simulink model "LKAS_AutoSave_DF_20220408_1006_SW62"  (R2018b)
settings: Solver=FixedStepDiscrete  StartTime=0.0  StopTime=10.0  FixedStep=0.01  RelTol=1e-3
undefined symbols (not defined in the file): LKA_CarWidth, LKA_SampleTime, LKA_StrRatio_C, LKA_Veh2CamL_C, LKA_Veh2CamW_C, LKA_WhlBaseL_C, LL_CompHdAg_C, LL_CompSWA_C, LL_CrvtPrvwT_C, LL_DesDvt_C, LL_DvtComp_C, LL_DvtPrvwT_C, LL_DvtSpdDet_vDvtSpdMin_C, LL_HandsOff_ExitTime, LL_HandsOff_TextTime, LL_HandsOff_WarnTime, LL_HdAgExT_C, LL_HdAgPrvwT_C, LL_LAccMax_C, LL_LAccRMax_C, LL_LDW_EarliestWarnLine_C, LL_LDW_LatestWarnLine_C, LL_LDWS_SUPPRESS_HEADING, LL_LFClb_TFC_FfCtlRatio_C, LL_LFClb_TFC_KdBalance_C, LL_LFClb_TFC_KdMaxSWA_C, LL_LFClb_TFC_KdV1_C, LL_LFClb_TFC_KdV2_C, LL_LFClb_TFC_KdVehSpdLwr_C, LL_LFClb_TFC_KdVehSpdUpr_C, LL_LFClb_TFC_Ki_C, LL_LFClb_TFC_KiMaxSWA_C, LL_LFClb_TFC_Kp_C, LL_LFClb_TFC_KpKlat_C, LL_LFClb_TFC_KpV1_C, LL_LFClb_TFC_KpV2_C, LL_LFClb_TFC_KpVehSpdLwr_C, LL_LFClb_TFC_KpVehSpdUpr_C, LL_LFClb_TFC_PrvwT_C, LL_LKA_EarliestWarnLine_C, LL_LKA_LatestWarnLine_C, LL_LKAExPrcs_ExitC0Dvt, LL_LKAExPrcs_ExitC0Swt, LL_LKAExPrcs_tiExitDelayTime3, LL_LKAExPrcs_tiExitTime1, LL_LKAExPrcs_tiExitTime2, LL_LKAExPrcs_tiExitTime3, LL_LKAS_OUT_OF_CONTROL_LAT_VEL, LL_LKAS_OUT_OF_CONTROL_TTLC, LL_LKASWASyn_M0, LL_LKASWASyn_M1, LL_LKASWASyn_M2, LL_LKASWASyn_M3D, LL_LKASWASyn_M3K_DT, LL_LKASWASyn_M3K_MSD, LL_LKASWASyn_M4K, LL_LKASWASyn_SWAaddMax, LL_LKASWASyn_T2, LL_LKASWASyn_tiTrqSwaRtTime, LL_LKASWASyn_tiTrqSwaTime ... (+47)
libraries: simulink x234, canmsglib x6, dspstat3 x3, simulink_extras x1
(part 8 of 16)

== system LKAS_AutoSave_DF_20220408_1006_SW62/LKAS/LL/LLOn/LKA/Lane Following (LF)/Trajectory Following Control (TFC) ==
  TFC_bsPrvwInfo : Inport
  TFC_bsInInfoSyn : Inport  Port=2
  TFC_bsTFCClb : Inport  Port=3
  Bus Selector1 : BusSelector  OutputSignals=bsLKAClb.LL_TFCClb.LL_LFClb_TFC_PrvwT_C,bsLKAClb.LL_TFCClb.LL_LFClb_TFC_KpKlat_C,bsLKAClb.LL_TFCClb.LL_LFClb_TFC_KpVehSpdLwr_C,bsLKAClb.LL_TFCClb.LL_LFClb_TFC_KpVehSpdUpr_C,bsLKAClb.LL_TFCClb.LL_LFClb_TFC_KpV1_C,bsLKAClb.LL_TFCClb.LL_LFClb_TFC_KpV2_C,bsLKAClb.LL_TFCClb.LL_LFClb_TFC_Kp_C,bsLKAClb.LL_TFCClb.LL_LFClb_TFC_KiMaxSWA_C,bsLKAClb.LL_TFCClb.LL_LFClb_TFC_Ki_C,bsLKAClb.LL_TFCClb.LL_LFClb_TFC_KdMaxSWA_C,bsLKAClb.LL_TFCClb.LL_LFClb_TFC_KdBalance_C,bsLKAClb.LL_TFCClb.LL_LFClb_TFC_KdVehSpdLwr_C,bsLKAClb.LL_TFCClb.LL_LFClb_TFC_KdVehSpdUpr_C,bsLKAClb.LL_TFCClb.LL_LFClb_TFC_KdV1_C,bsLKAClb.LL_TFCClb.LL_LFClb_TFC_KdV2_C,bsConstantClb.LKA_CarWidth,bsLKAClb.LL_TFCClb.LL_LFClb_TFC_FfCtlRatio_C,bsConstantClb.LKA_WhlBaseL_C,bsConstantClb.LKA_StrRatio_C
  Bus Selector2 : BusSelector  OutputSignals=lPrvwDvtMean (signal 1),phiPrvwHdAgMean (signal 2),crPrvwCrvtMean (signal 3),LaneWidth (signal 4),PrvwZMean (signal 5),crPrvwCrvtMean (signal 6)
  Bus Selector3 : BusSelector  OutputSignals=bsLaneInfo.bsL0Info,bsLaneInfo.bsR0Info,bsVehMovInfo.ESC_VehSpd
  Feedback Control (FbCtl) : Subsystem
  Feedforward Control (FfCtl) : Subsystem
  TFC_phiFfSWACmd : Outport
  TFC_phiPropSWACmd : Outport  Port=2
  TFC_phiIntegSWACmd : Outport  Port=3
  TFC_phiDiffSWACmd : Outport  Port=4
  wires:
  Bus Selector2/6 -> Feedback Control (FbCtl)/9(PrvwCrvtMean)  "<crPrvwCrvtMean (signal 6)>"
  Bus Selector2/5 -> Feedback Control (FbCtl)/8(PrvwZMean)  "<PrvwZMean (signal 5)>"
  Bus Selector2/2 -> Feedback Control (FbCtl)/5(FbCtl_PrvwHdAg)  "<phiPrvwHdAgMean (signal 2)>"
  Bus Selector1/19 -> Feedforward Control (FfCtl)/5(FfCtl_rTraRatio_C)  "<LKA_StrRatio_C>"
  Bus Selector1/18 -> Feedforward Control (FfCtl)/4(FfCtl_lWhlBase_SY)  "<LKA_WhlBaseL_C>"
  Bus Selector1/11 -> Feedback Control (FbCtl)/20(FbCtl_KdBalance)  "<LL_LFClb_TFC_KdBalance_C>"
  Bus Selector1/10 -> Feedback Control (FbCtl)/19(FbCtl_KdMaxSWA)  "<LL_LFClb_TFC_KdMaxSWA_C>"
  Feedback Control (FbCtl)/2(FbCtl_phiFbIntegCtlSWA) -> TFC_phiIntegSWACmd/1
  Bus Selector1/9 -> Feedback Control (FbCtl)/18(FbCtl_Ki_C)  "<LL_LFClb_TFC_Ki_C>"
  Bus Selector1/8 -> Feedback Control (FbCtl)/17(FbCtl_KiMaxSWA_C)  "<LL_LFClb_TFC_KiMaxSWA_C>"
  Bus Selector1/17 -> Feedforward Control (FfCtl)/1(FfCtl_FfCtlRatio_C)  "<LL_LFClb_TFC_FfCtlRatio_C>"
  Bus Selector1/6 -> Feedback Control (FbCtl)/15(FbCtl_KpV2_C1)  "<LL_LFClb_TFC_KpV2_C>"
  Bus Selector1/5 -> Feedback Control (FbCtl)/14(FbCtl_KpV1_C1)  "<LL_LFClb_TFC_KpV1_C>"
  Bus Selector1/4 -> Feedback Control (FbCtl)/13(FbCtl_KpVehSpdUpr_C)  "<LL_LFClb_TFC_KpVehSpdUpr_C>"
  Bus Selector1/3 -> Feedback Control (FbCtl)/12(FbCtl_KpVehSpdLwr_C)  "<LL_LFClb_TFC_KpVehSpdLwr_C>"
  Bus Selector3/3 -> Feedback Control (FbCtl)/3(FbCtl_VehSpd), Feedforward Control (FfCtl)/2(FfCtl_vVehSpd)  "<ESC_VehSpd>"
  Bus Selector1/2 -> Feedback Control (FbCtl)/11(FbCtl_KpKlat_C)  "<LL_LFClb_TFC_KpKlat_C>"
  Bus Selector1/1 -> Feedback Control (FbCtl)/10(FbCtl_PrvwT_C)  "<LL_LFClb_TFC_PrvwT_C>"
  TFC_bsTFCClb/1 -> Bus Selector1/1
  Bus Selector2/1 -> Feedback Control (FbCtl)/4(FbCtl_PrvwDvt)  "<lPrvwDvtMean (signal 1)>"
  TFC_bsPrvwInfo/1 -> Bus Selector2/1  "bsPrvwInfo"
  Feedback Control (FbCtl)/1(FbCtl_phiFbPropCtlSWA) -> TFC_phiPropSWACmd/1
  Feedforward Control (FfCtl)/1(FfCtl_phiFfSWA) -> TFC_phiFfSWACmd/1  "phiFfSWA"
  Bus Selector2/3 -> Feedback Control (FbCtl)/6(FbCtl_PrvwCrvt), Feedforward Control (FfCtl)/3(FfCtl_crPrvwCrvt)  "<crPrvwCrvtMean (signal 3)>"
  TFC_bsInInfoSyn/1 -> Bus Selector3/1
  Bus Selector3/1 -> Feedback Control (FbCtl)/1(FbCtl_bsL0Info)  "<bsL0Info>"
  Bus Selector3/2 -> Feedback Control (FbCtl)/2(FbCtl_bsR0Info)  "<bsR0Info>"
  Feedback Control (FbCtl)/3(FbCtl_phiFbDiffCtlSWA) -> TFC_phiDiffSWACmd/1
  Bus Selector1/7 -> Feedback Control (FbCtl)/16(FbCtl_Kp_C)  "<LL_LFClb_TFC_Kp_C>"
  Bus Selector1/12 -> Feedback Control (FbCtl)/21(FbCtl_KdVehSpdLwr_C)  "<LL_LFClb_TFC_KdVehSpdLwr_C>"
  Bus Selector1/13 -> Feedback Control (FbCtl)/22(FbCtl_KdVehSpdUpr_C)  "<LL_LFClb_TFC_KdVehSpdUpr_C>"
  Bus Selector1/14 -> Feedback Control (FbCtl)/23(FbCtl_KdV1_C)  "<LL_LFClb_TFC_KdV1_C>"
  Bus Selector1/15 -> Feedback Control (FbCtl)/24(FbCtl_KdV2_C)  "<LL_LFClb_TFC_KdV2_C>"
  Bus Selector2/4 -> Feedback Control (FbCtl)/7(FbCtl_LaneWidth)  "<LaneWidth (signal 4)>"
  Bus Selector1/16 -> Feedback Control (FbCtl)/25(FbCtl_CarWidth)  "<LKA_CarWidth>"

== system LKAS_AutoSave_DF_20220408_1006_SW62/LKAS/LL/LLOn/LKA/Plan To LaneFollowing (PTLF)/InsideJudge ==
  Flg : Inport
  Crvt : Inport  Port=2
  Compare To Constant : simulink/Logic and Bit Operations/Compare To Constant  relop===  const=1  OutDataTypeStr=boolean
  Compare To Constant1 : simulink/Logic and Bit Operations/Compare To Constant  relop===  const=2  OutDataTypeStr=boolean
  Constant : Constant  Value=0.001  OutDataTypeStr=single
  Constant3 : Constant  Value=-0.001  OutDataTypeStr=single
  Logical Operator : Logic  AllPortsSameDT=off  OutDataTypeStr=boolean
  Logical Operator1 : Logic  AllPortsSameDT=off  OutDataTypeStr=boolean
  Logical Operator2 : Logic  Operator=OR  AllPortsSameDT=off  OutDataTypeStr=boolean
  Relational Operator : RelationalOperator  OutDataTypeStr=boolean  RndMeth=Simplest
  Relational Operator1 : RelationalOperator  Operator=<=  OutDataTypeStr=boolean  RndMeth=Simplest
  Out1 : Outport
  wires:
  Crvt/1 -> Relational Operator/1, Relational Operator1/1
  Logical Operator2/1 -> Out1/1
  Constant3/1 -> Relational Operator1/2
  Relational Operator1/1 -> Logical Operator1/2  "LeftCrvt"
  Constant/1 -> Relational Operator/2
  Compare To Constant1/1 -> Logical Operator/1  "RightActive"
  Relational Operator/1 -> Logical Operator/2  "RightCrvt"
  Flg/1 -> Compare To Constant/1, Compare To Constant1/1
  Logical Operator/1 -> Logical Operator2/2
  Logical Operator1/1 -> Logical Operator2/1
  Compare To Constant/1 -> Logical Operator1/1  "LeftActive"

== system LKAS_AutoSave_DF_20220408_1006_SW62/LKAS/LL/LLOn/LKA/Plan To LaneFollowing (PTLF)/InsideJudge1 ==
  Flg : Inport
  HdAgLft : Inport  Port=2
  HdAgRgt : Inport  Port=3
  T1 : Inport  Port=4
  Plan : Inport  Port=5
  Time : Inport  Port=6
  If : If  IfExpression=u1 == 1  ElseIfExpressions=u1 == 2
  If Action Subsystem : Subsystem  TreatAsAtomicUnit=on
  If Action Subsystem1 : Subsystem  TreatAsAtomicUnit=on
  If Action Subsystem2 : Subsystem  TreatAsAtomicUnit=on
  Merge : Merge  Inputs=3  InitialOutput=1
  Merge1 : Merge  Inputs=3  InitialOutput=0
  T1_1 : Outport
  Plan_1 : Outport  Port=2
  wires:
  Time/1 -> If Action Subsystem/4(Time), If Action Subsystem1/4(Time)
  Merge1/1 -> Plan_1/1
  Merge/1 -> T1_1/1
  HdAgRgt/1 -> If Action Subsystem1/3(HdAgRgt)
  Plan/1 -> If Action Subsystem2/2(Plan), If Action Subsystem1/2(Plan), If Action Subsystem/2(Plan)
  T1/1 -> If Action Subsystem2/1(T1), If Action Subsystem1/1(T1), If Action Subsystem/1(T1)
  If Action Subsystem2/2(Plan_1) -> Merge1/3
  If Action Subsystem1/2(Plan_1) -> Merge1/2
  If Action Subsystem/2(Plan_1) -> Merge1/1
  If Action Subsystem2/1(T1_1) -> Merge/3
  If Action Subsystem1/1(T1_1) -> Merge/2
  If Action Subsystem/1(T1_1) -> Merge/1
  HdAgLft/1 -> If Action Subsystem/3(HdAgLft)
  If/3 -> If Action Subsystem2/Action
  If/2 -> If Action Subsystem1/Action
  If/1 -> If Action Subsystem/Action
  Flg/1 -> If/1

== system LKAS_AutoSave_DF_20220408_1006_SW62/LKAS/LL/LLOn/LKA/Plan To LaneFollowing (PTLF)/LowPass ==
  T : Inport
  u : Inport  Port=2
  dT : Inport  Port=3
  Add : Sum  Inputs=+-
  Add1 : Sum
  Add2 : Sum  OutDataTypeStr=single
  Divide : Product  Inputs=*/
  Divide1 : Product  Inputs=**
  Memory3 : Memory  InheritSampleTime=on
  SWACmdSyn_tiSmplT_C4 : Constant  OutDataTypeStr=single
  Saturation : Saturate  UpperLimit=50  LowerLimit=0
      settings: AttributesFormatString="Min = %<LowerLimit>  Max = %<UpperLimit>"
  Switch : Switch  Criteria=u2 > Threshold  Threshold=30
  Unit Delay : UnitDelay  SampleTime=-1
  y : Outport
  wires:
  T/1 -> Divide/2
  dT/1 -> Divide/1
  u/1 -> Switch/3, Add/1
  Divide/1 -> Divide1/1
  Add/1 -> Divide1/2
  Divide1/1 -> Add1/1
  Unit Delay/1 -> Add/2, Add1/2
  Add1/1 -> Switch/1
  SWACmdSyn_tiSmplT_C4/1 -> Add2/1
  Add2/1 -> Saturation/1
  Saturation/1 -> Switch/2, Memory3/1
  Memory3/1 -> Add2/2
  Switch/1 -> y/1, Unit Delay/1

== system LKAS_AutoSave_DF_20220408_1006_SW62/LKAS/LL/LLOn/LKA/Plan To LaneFollowing (PTLF)/TickTime (TTime) ==
  Add2 : Sum  OutDataTypeStr=single
  Memory3 : Memory  InheritSampleTime=on
  Saturation : Saturate  UpperLimit=50  LowerLimit=0
      settings: AttributesFormatString="Min = %<LowerLimit>  Max = %<UpperLimit>"
  Out1 : Outport
  wires:
  [LKA_SampleTime] -> Add2/1
  Saturation/1 -> Memory3/1, Out1/1
  Memory3/1 -> Add2/2
  Add2/1 -> Saturation/1

== system LKAS_AutoSave_DF_20220408_1006_SW62/LKAS/LL/LLOn/LKA/Plan To LaneFollowing (PTLF)/TimeGain ==
  Time : Inport
  T1 : Inport  Port=2
  TFC : Inport  Port=3
  Add1 : Sum
  Add2 : Sum  Inputs=+-
  Add3 : Sum  Inputs=-+
  Constant1 : Constant  Value=0  OutDataTypeStr=single
  Constant4 : Constant  OutDataTypeStr=single
  Divide : Product  Inputs=*/
  Divide8 : Product  Inputs=**
  Saturation4 : Saturate  UpperLimit=1  LowerLimit=0
      settings: AttributesFormatString="Min = %<LowerLimit>  Max = %<UpperLimit>"
  Out1 : Outport
  wires:
  Add3/1 -> Divide8/1
  Constant4/1 -> Add3/2
  Add2/1 -> Divide/1
  Divide/1 -> Saturation4/1
  Time/1 -> Add2/1
  T1/1 -> Add2/2
  TFC/1 -> Divide/2
  Add1/1 -> Out1/1
  Divide8/1 -> Add1/2
  Constant1/1 -> Add3/1, Add1/1
  Saturation4/1 -> Divide8/2

== system LKAS_AutoSave_DF_20220408_1006_SW62/LKAS/LL/LLOn/LKA Input Processing (LKAInP)/Deviation Calculation (Dvt)/Left Front Conner Deviation Calculation (LFCDvtCalc) ==
  LFCDvtCalc_bsHdAgInfo : Inport
  LFCDvtCalc_lDvt : Inport  Port=2
  LFCDvtCalc_bsLLClb : Inport  Port=3
  Add1 : Sum  OutDataTypeStr=single
  Add5 : Sum  OutDataTypeStr=single
  Bus Selector : BusSelector  OutputSignals=bsConstantClb.LKA_Veh2CamW_C,bsConstantClb.LKA_Veh2CamL_C
  Cos2 : Trigonometry  Operator=cos
  Divide : Product  Inputs=**
  Divide1 : Product  Inputs=**
  Gain1 : Gain  Gain=-1  OutDataTypeStr=single
  Sin : Trigonometry
  DvtCalc_lLftDvt : Outport
  wires:
  Add5/1 -> Gain1/1
  Add1/1 -> Divide/1
  Divide1/1 -> Add5/2
  Divide/1 -> Add5/1
  Sin/1 -> Divide1/2
  Cos2/1 -> Divide/2
  Gain1/1 -> DvtCalc_lLftDvt/1
  LFCDvtCalc_bsHdAgInfo/1 -> Sin/1, Cos2/1
  Bus Selector/2 -> Divide1/1  "<LKA_Veh2CamL_C>"
  LFCDvtCalc_bsLLClb/1 -> Bus Selector/1
  Bus Selector/1 -> Add1/2  "<LKA_Veh2CamW_C>"
  LFCDvtCalc_lDvt/1 -> Add1/1

== system LKAS_AutoSave_DF_20220408_1006_SW62/LKAS/LL/LLOn/LKA Input Processing (LKAInP)/Deviation Calculation (Dvt)/Right Front Conner Deviation Calculation (RFCDvtCalc) ==
  RFCDvtCalc_lDvt : Inport
  RFCDvtCalc_bsHdAgInfo : Inport  Port=2
  RFCDvtCalc_bsLLClb : Inport  Port=3
  Add1 : Sum  Inputs=+-  OutDataTypeStr=single
  Add5 : Sum  OutDataTypeStr=single
  Bus Selector1 : BusSelector  OutputSignals=bsConstantClb.LKA_Veh2CamW_C,bsConstantClb.LKA_Veh2CamL_C
  Cos2 : Trigonometry  Operator=cos
  Divide : Product  Inputs=**
  Divide1 : Product  Inputs=**
  Sin : Trigonometry
  DvtCalc_lRgtDvt : Outport
  wires:
  RFCDvtCalc_bsLLClb/1 -> Bus Selector1/1
  Divide/1 -> Add5/1
  Add1/1 -> Divide/1
  Cos2/1 -> Divide/2
  RFCDvtCalc_bsHdAgInfo/1 -> Sin/1, Cos2/1
  Divide1/1 -> Add5/2
  Sin/1 -> Divide1/2
  Add5/1 -> DvtCalc_lRgtDvt/1
  Bus Selector1/2 -> Divide1/1  "<LKA_Veh2CamL_C>"
  Bus Selector1/1 -> Add1/2  "<LKA_Veh2CamW_C>"
  RFCDvtCalc_lDvt/1 -> Add1/1

== system LKAS_AutoSave_DF_20220408_1006_SW62/LKAS/LL/LLOn/LKA Input Processing (LKAInP)/Previewed Curvature Calculation (PrCrvt)/Curvature Ahead of Left Lane Line (CrvtAhdLft) ==
  CrvtAhdLft_bsL0Info : Inport
  CrvtAhdLft_lPrvwDstZ : Inport  Port=2
  Add : Sum  AccumDataTypeStr=single
  Bus Selector : BusSelector  OutputSignals=L0_C2,L0_C3
  Gain : Gain  Gain=2  OutDataTypeStr=single
  Gain1 : Gain  Gain=6  OutDataTypeStr=single
  Product : Product  OutDataTypeStr=single  RndMeth=Zero
  CrvtAhdLft_crCrvtAhdLft : Outport
  wires:
  CrvtAhdLft_bsL0Info/1 -> Bus Selector/1
  Bus Selector/2 -> Gain1/1  "<L0_C3>"
  CrvtAhdLft_lPrvwDstZ/1 -> Product/2
  Bus Selector/1 -> Gain/1  "<L0_C2>"
  Gain1/1 -> Product/1
  Gain/1 -> Add/1
  Product/1 -> Add/2
  Add/1 -> CrvtAhdLft_crCrvtAhdLft/1

== system LKAS_AutoSave_DF_20220408_1006_SW62/LKAS/LL/LLOn/LKA Input Processing (LKAInP)/Previewed Curvature Calculation (PrCrvt)/Curvature Ahead of Left Lane Line (CrvtAhdLft)1 ==
  CrvtAhdRgt_lPrvwDstZ : Inport
  CrvtAhdRgt_bsR0Info : Inport  Port=2
  Add : Sum  AccumDataTypeStr=single
  Bus Selector : BusSelector  OutputSignals=R0_C2,R0_C3
  Gain : Gain  Gain=2  OutDataTypeStr=single
  Gain1 : Gain  Gain=6  OutDataTypeStr=single
  Product : Product  OutDataTypeStr=single  RndMeth=Zero
  CrvtAhdRgt_crCrvtAhdRgt : Outport
  wires:
  CrvtAhdRgt_bsR0Info/1 -> Bus Selector/1
  Bus Selector/2 -> Gain1/1  "<R0_C3>"
  CrvtAhdRgt_lPrvwDstZ/1 -> Product/2
  Bus Selector/1 -> Gain/1  "<R0_C2>"
  Gain1/1 -> Product/1
  Gain/1 -> Add/1
  Product/1 -> Add/2
  Add/1 -> CrvtAhdRgt_crCrvtAhdRgt/1

== system LKAS_AutoSave_DF_20220408_1006_SW62/LKAS/LL/LLOn/LKA Input Processing (LKAInP)/Previewed Curvature Calculation (PrCrvt)/Lane Information Selection (LaneInfoSel) ==
  LaneInfoSel_stLKAActvFlg : Inport
  LaneInfoSel_facmLftLane : Inport  Port=2
  LaneInfoSel_facmRgtLane : Inport  Port=3
  If : If  IfExpression=u1==1  ElseIfExpressions=u1==2
  If Action Subsystem1 : Subsystem  TreatAsAtomicUnit=on
  If Action Subsystem2 : Subsystem  TreatAsAtomicUnit=on
  If Action Subsystem3 : Subsystem  TreatAsAtomicUnit=on
  Merge : Merge  Inputs=3
  LaneInfoSel_facmActvLane : Outport
  wires:
  LaneInfoSel_facmLftLane/1 -> If Action Subsystem2/1(In1), If Action Subsystem3/1(In1)
  LaneInfoSel_facmRgtLane/1 -> If Action Subsystem1/1(In1), If Action Subsystem3/2(In2)
  LaneInfoSel_stLKAActvFlg/1 -> If/1
  If/1 -> If Action Subsystem2/Action
  If Action Subsystem2/1(Out1) -> Merge/1
  Merge/1 -> LaneInfoSel_facmActvLane/1
  If/2 -> If Action Subsystem1/Action
  If Action Subsystem1/1(Out1) -> Merge/2
  If Action Subsystem3/1(Out1) -> Merge/3
  If/3 -> If Action Subsystem3/Action

== system LKAS_AutoSave_DF_20220408_1006_SW62/LKAS/LL/LLOn/LKA Input Processing (LKAInP)/Previewed Curvature Calculation (PrCrvt)/Z Calculation (ZCalc) ==
  ZCalc_vVehSpd : Inport
  ZCalc_tiCrvtPrvwT_C : Inport  Port=2
  Divide : Product  Inputs=**  OutDataTypeStr=single
  kph to mps : Gain  Gain=1/3.6  OutDataTypeStr=single
  ZCalc_lPrvwDstZ : Outport
  wires:
  ZCalc_vVehSpd/1 -> kph to mps/1
  ZCalc_tiCrvtPrvwT_C/1 -> Divide/2
  kph to mps/1 -> Divide/1
  Divide/1 -> ZCalc_lPrvwDstZ/1

== system LKAS_AutoSave_DF_20220408_1006_SW62/LKAS/LL/LLOn/LKA Input Processing (LKAInP)/Previewed Deviation Calculation (PrDvt)/Previewed Deviation of Left Lane Line (PrvwDvtLft) ==
  PrdcDvtLft_bsL0Info : Inport
  PrdcDvtLft_lPrvwDstZ : Inport  Port=2
  Add : Sum  Inputs=++++  AccumDataTypeStr=single
  Bus Selector : BusSelector  OutputSignals=L0_C0,L0_C1,L0_C2,L0_C3
  Product : Product  OutDataTypeStr=single  RndMeth=Zero
  Product3 : Product  OutDataTypeStr=single  RndMeth=Zero
  Product4 : Product  OutDataTypeStr=single  RndMeth=Zero
  Z*Z : Product  OutDataTypeStr=single  RndMeth=Zero
  Z*Z*Z : Product  OutDataTypeStr=single  RndMeth=Zero
  PrvwDvtLft_lPrvwDvtLft : Outport
  wires:
  Add/1 -> PrvwDvtLft_lPrvwDvtLft/1
  PrdcDvtLft_bsL0Info/1 -> Bus Selector/1
  PrdcDvtLft_lPrvwDstZ/1 -> Z*Z*Z/1, Z*Z/1, Product/2, Z*Z/2
  Bus Selector/2 -> Product/1  "<L0_C1>"
  Product/1 -> Add/2
  Bus Selector/1 -> Add/1  "<L0_C0>"
  Product3/1 -> Add/3
  Bus Selector/3 -> Product3/1  "<L0_C2>"
  Bus Selector/4 -> Product4/1  "<L0_C3>"
  Product4/1 -> Add/4
  Z*Z*Z/1 -> Product4/2
  Z*Z/1 -> Product3/2, Z*Z*Z/2

== system LKAS_AutoSave_DF_20220408_1006_SW62/LKAS/LL/LLOn/LKA Input Processing (LKAInP)/Previewed Deviation Calculation (PrDvt)/Previewed Deviation of Right Lane Line (PrvwDvtRgt) ==
  PrdcDvtRgt_lPrvwDstZ : Inport
  PrdcDvtRgt_bsR0Info : Inport  Port=2
  Add : Sum  Inputs=++++  AccumDataTypeStr=single
  Bus Selector : BusSelector  OutputSignals=R0_C0,R0_C1,R0_C2,R0_C3
  Product : Product  OutDataTypeStr=single  RndMeth=Zero
  Product3 : Product  OutDataTypeStr=single  RndMeth=Zero
  Product4 : Product  OutDataTypeStr=single  RndMeth=Zero
  Z*Z : Product  OutDataTypeStr=single  RndMeth=Zero
  Z*Z*Z : Product  OutDataTypeStr=single  RndMeth=Zero
  PrvwDvtRgt_lPrvwDvtRgt : Outport
  wires:
  PrdcDvtRgt_bsR0Info/1 -> Bus Selector/1
  PrdcDvtRgt_lPrvwDstZ/1 -> Z*Z*Z/1, Z*Z/1, Product/2, Z*Z/2
  Bus Selector/2 -> Product/1  "<R0_C1>"
  Product/1 -> Add/2
  Add/1 -> PrvwDvtRgt_lPrvwDvtRgt/1
  Bus Selector/1 -> Add/1  "<R0_C0>"
  Product3/1 -> Add/3
  Bus Selector/3 -> Product3/1  "<R0_C2>"
  Bus Selector/4 -> Product4/1  "<R0_C3>"
  Product4/1 -> Add/4
  Z*Z*Z/1 -> Product4/2
  Z*Z/1 -> Product3/2, Z*Z*Z/2

== system LKAS_AutoSave_DF_20220408_1006_SW62/LKAS/LL/LLOn/LKA Input Processing (LKAInP)/Previewed Deviation Calculation (PrDvt)/Z Calculation (ZCalc) ==
  ZCalc_vVehSpd : Inport
  ZCalc_tiDvtPrvwT_C : Inport  Port=2
  Divide : Product  Inputs=**  OutDataTypeStr=single
  kph to mps : Gain  Gain=1/3.6  OutDataTypeStr=single
  ZCalc_lPrvwDstZ : Outport
  wires:
  ZCalc_vVehSpd/1 -> kph to mps/1
  kph to mps/1 -> Divide/1
  Divide/1 -> ZCalc_lPrvwDstZ/1
  ZCalc_tiDvtPrvwT_C/1 -> Divide/2

== system LKAS_AutoSave_DF_20220408_1006_SW62/LKAS/LL/LLOn/LKA Input Processing (LKAInP)/Previewed Heading Angle Calculation (PrHdAg)/Perdicted Heading Angle from Right Lane Line (PrdcHdAgRgt)1 ==
  PrdcHdAgRgt_lPrvwDstZ : Inport
  PrdcHdAgRgt_bsR0Info : Inport  Port=2
  Add : Sum  Inputs=+++  AccumDataTypeStr=single
  Bus Selector : BusSelector  OutputSignals=R0_C1,R0_C2,R0_C3
  Gain : Gain  Gain=2  OutDataTypeStr=single
  Gain1 : Gain  Gain=3  OutDataTypeStr=single
  Product3 : Product  OutDataTypeStr=single  RndMeth=Zero
  Product4 : Product  OutDataTypeStr=single  RndMeth=Zero
  Z*Z : Product  OutDataTypeStr=single  RndMeth=Zero
  PrdcHdAgRgt_phiPrdcHdAgRgt : Outport
  wires:
  Add/1 -> PrdcHdAgRgt_phiPrdcHdAgRgt/1
  PrdcHdAgRgt_bsR0Info/1 -> Bus Selector/1
  PrdcHdAgRgt_lPrvwDstZ/1 -> Z*Z/1, Product3/2, Z*Z/2
  Bus Selector/1 -> Add/1  "<R0_C1>"
  Product3/1 -> Add/2
  Bus Selector/2 -> Gain/1  "<R0_C2>"
  Bus Selector/3 -> Gain1/1  "<R0_C3>"
  Product4/1 -> Add/3
  Z*Z/1 -> Product4/2
  Gain/1 -> Product3/1
  Gain1/1 -> Product4/1

== system LKAS_AutoSave_DF_20220408_1006_SW62/LKAS/LL/LLOn/LKA Input Processing (LKAInP)/Previewed Heading Angle Calculation (PrHdAg)/Perdicted Heading Angle from Right Lane Line (PrvwTTLCHdAgLftTTLCRgt) ==
  PrdcHdAgRgt_lPrvwDstZ : Inport
  PrdcHdAgRgt_bsR0Info : Inport  Port=2
  Add : Sum  Inputs=+++  AccumDataTypeStr=single
  Bus Selector : BusSelector  OutputSignals=R0_C1,R0_C2,R0_C3
  Gain : Gain  Gain=2  OutDataTypeStr=single
  Gain1 : Gain  Gain=3  OutDataTypeStr=single
  Product3 : Product  OutDataTypeStr=single  RndMeth=Zero
  Product4 : Product  OutDataTypeStr=single  RndMeth=Zero
  Z*Z : Product  OutDataTypeStr=single  RndMeth=Zero
  PrdcHdAgRgt_phiPrdcHdAgRgt : Outport
  wires:
  Gain1/1 -> Product4/1
  Gain/1 -> Product3/1
  Z*Z/1 -> Product4/2
  Product4/1 -> Add/3
  Bus Selector/3 -> Gain1/1  "<R0_C3>"
  Bus Selector/2 -> Gain/1  "<R0_C2>"
  Product3/1 -> Add/2
  Bus Selector/1 -> Add/1  "<R0_C1>"
  PrdcHdAgRgt_lPrvwDstZ/1 -> Z*Z/2, Product3/2, Z*Z/1
  PrdcHdAgRgt_bsR0Info/1 -> Bus Selector/1
  Add/1 -> PrdcHdAgRgt_phiPrdcHdAgRgt/1

== system LKAS_AutoSave_DF_20220408_1006_SW62/LKAS/LL/LLOn/LKA Input Processing (LKAInP)/Previewed Heading Angle Calculation (PrHdAg)/Perdicted Heading Angle from Right Lane Line (PrvwTTLCHdAgRgtTTLCRgt) ==
  PrdcHdAgRgt_lPrvwDstZ : Inport
  PrdcHdAgRgt_bsR0Info : Inport  Port=2
  Add : Sum  Inputs=+++  AccumDataTypeStr=single
  Bus Selector : BusSelector  OutputSignals=R0_C1,R0_C2,R0_C3
  Gain : Gain  Gain=2  OutDataTypeStr=single
  Gain1 : Gain  Gain=3  OutDataTypeStr=single
  Product3 : Product  OutDataTypeStr=single  RndMeth=Zero
  Product4 : Product  OutDataTypeStr=single  RndMeth=Zero
  Z*Z : Product  OutDataTypeStr=single  RndMeth=Zero
  PrdcHdAgRgt_phiPrdcHdAgRgt : Outport
  wires:
  Add/1 -> PrdcHdAgRgt_phiPrdcHdAgRgt/1
  PrdcHdAgRgt_bsR0Info/1 -> Bus Selector/1
  PrdcHdAgRgt_lPrvwDstZ/1 -> Z*Z/1, Product3/2, Z*Z/2
  Bus Selector/1 -> Add/1  "<R0_C1>"
  Product3/1 -> Add/2
  Bus Selector/2 -> Gain/1  "<R0_C2>"
  Bus Selector/3 -> Gain1/1  "<R0_C3>"
  Product4/1 -> Add/3
  Z*Z/1 -> Product4/2
  Gain/1 -> Product3/1
  Gain1/1 -> Product4/1

== system LKAS_AutoSave_DF_20220408_1006_SW62/LKAS/LL/LLOn/LKA Input Processing (LKAInP)/Previewed Heading Angle Calculation (PrHdAg)/Predicted Heading Angle from Left Lane Line (PrdcHdAgtLft)1 ==
  PrdcHdAgtLft_bsL0Info : Inport
  PrdcHdAgtLft_lPrvwDstZ : Inport  Port=2
  Add : Sum  Inputs=+++  AccumDataTypeStr=single
  Bus Selector : BusSelector  OutputSignals=L0_C1,L0_C2,L0_C3
  Gain : Gain  Gain=2  OutDataTypeStr=single
  Gain1 : Gain  Gain=3  OutDataTypeStr=single
  Product3 : Product  OutDataTypeStr=single  RndMeth=Zero
  Product4 : Product  OutDataTypeStr=single  RndMeth=Zero
  Z*Z : Product  OutDataTypeStr=single  RndMeth=Zero
  PrdcHdAgtLft_phiPrdcHdAgLft : Outport
  wires:
  Add/1 -> PrdcHdAgtLft_phiPrdcHdAgLft/1
  PrdcHdAgtLft_bsL0Info/1 -> Bus Selector/1
  PrdcHdAgtLft_lPrvwDstZ/1 -> Z*Z/1, Product3/2, Z*Z/2
  Bus Selector/1 -> Add/1  "<L0_C1>"
  Product3/1 -> Add/2
  Bus Selector/2 -> Gain/1  "<L0_C2>"
  Bus Selector/3 -> Gain1/1  "<L0_C3>"
  Product4/1 -> Add/3
  Z*Z/1 -> Product4/2
  Gain/1 -> Product3/1
  Gain1/1 -> Product4/1

== system LKAS_AutoSave_DF_20220408_1006_SW62/LKAS/LL/LLOn/LKA Input Processing (LKAInP)/Previewed Heading Angle Calculation (PrHdAg)/Predicted Heading Angle from Left Lane Line (PrdcHdAgtLftTTLCLft) ==
  PrdcHdAgtLft_bsL0Info : Inport
  PrdcHdAgtLft_lPrvwDstZ : Inport  Port=2
  Add : Sum  Inputs=+++  AccumDataTypeStr=single
  Bus Selector : BusSelector  OutputSignals=L0_C1,L0_C2,L0_C3
  Gain : Gain  Gain=2  OutDataTypeStr=single
  Gain1 : Gain  Gain=3  OutDataTypeStr=single
  Product3 : Product  OutDataTypeStr=single  RndMeth=Zero
  Product4 : Product  OutDataTypeStr=single  RndMeth=Zero
  Z*Z : Product  OutDataTypeStr=single  RndMeth=Zero
  PrdcHdAgtLft_phiPrdcHdAgLft : Outport
  wires:
  Add/1 -> PrdcHdAgtLft_phiPrdcHdAgLft/1
  PrdcHdAgtLft_bsL0Info/1 -> Bus Selector/1
  PrdcHdAgtLft_lPrvwDstZ/1 -> Z*Z/1, Product3/2, Z*Z/2
  Bus Selector/1 -> Add/1  "<L0_C1>"
  Product3/1 -> Add/2
  Bus Selector/2 -> Gain/1  "<L0_C2>"
  Bus Selector/3 -> Gain1/1  "<L0_C3>"
  Product4/1 -> Add/3
  Z*Z/1 -> Product4/2
  Gain/1 -> Product3/1
  Gain1/1 -> Product4/1

== system LKAS_AutoSave_DF_20220408_1006_SW62/LKAS/LL/LLOn/LKA Input Processing (LKAInP)/Previewed Heading Angle Calculation (PrHdAg)/Predicted Heading Angle from Left Lane Line (PrvwTTLCHdAgRgtTTLCLft) ==
  PrdcHdAgtLft_bsL0Info : Inport
  PrdcHdAgtLft_lPrvwDstZ : Inport  Port=2
  Add : Sum  Inputs=+++  AccumDataTypeStr=single
  Bus Selector : BusSelector  OutputSignals=L0_C1,L0_C2,L0_C3
  Gain : Gain  Gain=2  OutDataTypeStr=single
  Gain1 : Gain  Gain=3  OutDataTypeStr=single
  Product3 : Product  OutDataTypeStr=single  RndMeth=Zero
  Product4 : Product  OutDataTypeStr=single  RndMeth=Zero
  Z*Z : Product  OutDataTypeStr=single  RndMeth=Zero
  PrdcHdAgtLft_phiPrdcHdAgLft : Outport
  wires:
  Gain1/1 -> Product4/1
  Gain/1 -> Product3/1
  Z*Z/1 -> Product4/2
  Product4/1 -> Add/3
  Bus Selector/3 -> Gain1/1  "<L0_C3>"
  Bus Selector/2 -> Gain/1  "<L0_C2>"
  Product3/1 -> Add/2
  Bus Selector/1 -> Add/1  "<L0_C1>"
  PrdcHdAgtLft_lPrvwDstZ/1 -> Z*Z/2, Product3/2, Z*Z/1
  PrdcHdAgtLft_bsL0Info/1 -> Bus Selector/1
  Add/1 -> PrdcHdAgtLft_phiPrdcHdAgLft/1

== system LKAS_AutoSave_DF_20220408_1006_SW62/LKAS/LL/LLOn/LKA Input Processing (LKAInP)/Previewed Heading Angle Calculation (PrHdAg)/Z Calculation (ZCalc) ==
  ZCalc_vVehSpd : Inport
  ZCalc_tiHdAgPrvwT_C : Inport  Port=2
  Divide : Product  Inputs=**  OutDataTypeStr=single
  kph to mps : Gain  Gain=1/3.6  OutDataTypeStr=single
  ZCalc_lPrvwDstZ : Outport
  wires:
  ZCalc_vVehSpd/1 -> kph to mps/1
  ZCalc_tiHdAgPrvwT_C/1 -> Divide/2
  Divide/1 -> ZCalc_lPrvwDstZ/1
  kph to mps/1 -> Divide/1

== system LKAS_AutoSave_DF_20220408_1006_SW62/LKAS/LL/LLOn/LKA Input Processing (LKAInP)/Previewed Heading Angle Calculation (PrHdAg)/Z Calculation (ZCalc)1 ==
  ZCalc_vVehSpd : Inport
  ZCalc_tiHdAgPrvwT_C : Inport  Port=2
  Divide : Product  Inputs=**  OutDataTypeStr=single
  kph to mps : Gain  Gain=1/3.6  OutDataTypeStr=single
  ZCalc_lPrvwDstZ : Outport
  wires:
  ZCalc_vVehSpd/1 -> kph to mps/1
  ZCalc_tiHdAgPrvwT_C/1 -> Divide/2
  Divide/1 -> ZCalc_lPrvwDstZ/1
  kph to mps/1 -> Divide/1

== system LKAS_AutoSave_DF_20220408_1006_SW62/LKAS/LL/LLOn/LKA Input Processing (LKAInP)/Steering Wheel Position Calculation (SWAPosCal)/Subsystem ==
  SWAIn : Inport
  LKA_SampleTime : Inport  Port=2
  Enable : EnablePort
      settings: AttributesFormatString=states = %<StatesWhenEnabling>
  Constant : Constant  Value=10  OutDataTypeStr=single
  LowPass : Subsystem
  Saturation : Saturate  UpperLimit=3  LowerLimit=-3
      settings: AttributesFormatString="Min = %<LowerLimit>  Max = %<UpperLimit>"
  SWAPos : Outport  InitialOutput=0
      settings: AttributesFormatString=%<OutputWhenDisabled> = %<InitialOutput>
  wires:
  Saturation/1 -> SWAPos/1
  LKA_SampleTime/1 -> LowPass/3(dT)
  Constant/1 -> LowPass/1(T)
  LowPass/1(y) -> Saturation/1  "SWAPos"
  SWAIn/1 -> LowPass/2(u)

== system LKAS_AutoSave_DF_20220408_1006_SW62/LKAS/LL/LLOn/LKA Input Processing (LKAInP)/Steering Wheel Position Calculation (SWAPosCal)/Subsystem1 ==
  L0 : Inport
  R0 : Inport  Port=2
  VehSpd : Inport  Port=3
  SWA : Inport  Port=4
  LKA_SampleTime : Inport  Port=5
  Abs{2,4..7} (5 alike) : Abs
  Bus Selector : BusSelector  OutputSignals=L0_C1,L0_C2,L0_Q
  Bus Selector1 : BusSelector  OutputSignals=R0_C1,R0_C2,R0_Q
  Compare To Constant : simulink/Logic and Bit Operations/Compare To Constant  relop===  const=3.0  OutDataTypeStr=boolean
  Compare To Constant1 : simulink/Logic and Bit Operations/Compare To Constant  relop===  const=3.0  OutDataTypeStr=boolean
  Constant : Constant  Value=0.0001  OutDataTypeStr=single
  Constant1 : Constant  Value=0.008  OutDataTypeStr=single
  Constant3 : Constant  Value=2  OutDataTypeStr=single
  Constant4 : Constant  Value=35  OutDataTypeStr=single
  Constant5 : Constant  Value=4  OutDataTypeStr=single
  Divide : Product  Inputs=*/
  Logical Operator : Logic  AllPortsSameDT=off  OutDataTypeStr=boolean
  Logical Operator1 : Logic  AllPortsSameDT=off  OutDataTypeStr=boolean
  Logical Operator3 : Logic  Inputs=5  AllPortsSameDT=off  OutDataTypeStr=boolean
  Logical Operator4 : Logic  AllPortsSameDT=off  OutDataTypeStr=boolean
  Relational Operator{,1..3,7} (5 alike) : RelationalOperator  Operator=<=  OutDataTypeStr=boolean  RndMeth=Simplest
  Relational Operator6 : RelationalOperator  OutDataTypeStr=boolean  RndMeth=Simplest
  Subsystem : Subsystem
  Flg : Outport
  wires:
  LKA_SampleTime/1 -> Divide/2
  Relational Operator/1 -> Logical Operator/1
  Divide/1 -> Subsystem/2(In1)
  Bus Selector/2 -> Abs4/1  "<L0_C2>"
  Logical Operator4/1 -> Logical Operator3/3
  Bus Selector1/1 -> Abs7/1  "<R0_C1>"
  Bus Selector/1 -> Abs6/1  "<L0_C1>"
  Subsystem/1(Out) -> Flg/1
  Constant5/1 -> Relational Operator7/2
  Logical Operator/1 -> Logical Operator3/2
  SWA/1 -> Abs2/1
  Relational Operator3/1 -> Logical Operator1/2
  Relational Operator1/1 -> Logical Operator/2
  Abs5/1 -> Relational Operator1/1
  Bus Selector1/2 -> Abs5/1  "<R0_C2>"
  Relational Operator7/1 -> Logical Operator3/5
  Compare To Constant/1 -> Logical Operator4/1
  Abs6/1 -> Relational Operator2/1
  Constant4/1 -> Relational Operator6/2
  VehSpd/1 -> Relational Operator6/1
  Logical Operator3/1 -> Subsystem/1(In), Subsystem/Enable  "SWA"
  Constant3/1 -> Divide/1
  Abs4/1 -> Relational Operator/1
  Constant/1 -> Relational Operator/2, Relational Operator1/2
  Constant1/1 -> Relational Operator2/2, Relational Operator3/2
  Abs7/1 -> Relational Operator3/1
  Relational Operator6/1 -> Logical Operator3/4
  Compare To Constant1/1 -> Logical Operator4/2
  Relational Operator2/1 -> Logical Operator1/1
  Bus Selector1/3 -> Compare To Constant1/1  "<R0_Q>"
  Abs2/1 -> Relational Operator7/1
  Bus Selector/3 -> Compare To Constant/1  "<L0_Q>"
  Logical Operator1/1 -> Logical Operator3/1
  R0/1 -> Bus Selector1/1
  L0/1 -> Bus Selector/1

== system LKAS_AutoSave_DF_20220408_1006_SW62/LKAS/LL/LLOn/LKA Input Processing (LKAInP)/Under The Limit (UndrLim)/Steering Wheel Angel Max (SWAMax) ==
  SWAMax_vVehSpd : Inport
  SWAMax_aLAcc_C : Inport  Port=2
  LKA_StrRatio_C : Inport  Port=3
  LKA_WhlBaseL_C : Inport  Port=4
  Constant : Constant  Value=0.09  OutDataTypeStr=single
  Divide1 : Product  Inputs=*/
  MATLAB Function : MATLAB Function  TreatAsAtomicUnit=on
  Saturation1 : Saturate  UpperLimit=0.0117  LowerLimit=0.00237
      settings: AttributesFormatString="Min = %<LowerLimit>  Max = %<UpperLimit>"
  Saturation3 : Saturate  UpperLimit=150  LowerLimit=60
      settings: AttributesFormatString="Min = %<LowerLimit>  Max = %<UpperLimit>"
  kph To mps : Gain  Gain=1/3.6  OutDataTypeStr=single
  SWAMax_phiSWAMax : Outport
  wires:
  Saturation3/1 -> Divide1/2  "Vx"
  Constant/1 -> Divide1/1
  MATLAB Function/1(SWAmax) -> SWAMax_phiSWAMax/1
  SWAMax_aLAcc_C/1 -> MATLAB Function/2(ax)
  Saturation1/1 -> MATLAB Function/5(K)
  Divide1/1 -> Saturation1/1
  SWAMax_vVehSpd/1 -> kph To mps/1, Saturation3/1
  kph To mps/1 -> MATLAB Function/1(v)
  LKA_WhlBaseL_C/1 -> MATLAB Function/4(L)
  LKA_StrRatio_C/1 -> MATLAB Function/3(i)

== system LKAS_AutoSave_DF_20220408_1006_SW62/LKAS/LL/LLOn/LKA Input Processing (LKAInP)/Under The Limit (UndrLim)/Steering Wheel Angel Rate Max (SWARMax) ==
  SWARateMax_vVehSpd : Inport
  SWARateMax_aLAccR_C : Inport  Port=2
  LKA_StrRatio_C : Inport  Port=3
  LKA_WhlBaseL_C : Inport  Port=4
  Constant : Constant  Value=0.09  OutDataTypeStr=single
  Divide1 : Product  Inputs=*/
  MATLAB Function : MATLAB Function  TreatAsAtomicUnit=on
  Saturation1 : Saturate  UpperLimit=0.0117  LowerLimit=0.00237
      settings: AttributesFormatString="Min = %<LowerLimit>  Max = %<UpperLimit>"
  Saturation3 : Saturate  UpperLimit=150  LowerLimit=60
      settings: AttributesFormatString="Min = %<LowerLimit>  Max = %<UpperLimit>"
  kph To mps : Gain  Gain=1/3.6  OutDataTypeStr=single
  SWARMax_dphiSWARMax : Outport
  wires:
  Saturation3/1 -> Divide1/2  "Vx"
  Constant/1 -> Divide1/1
  SWARateMax_aLAccR_C/1 -> MATLAB Function/2(dax)
  Saturation1/1 -> MATLAB Function/5(K)
  Divide1/1 -> Saturation1/1
  SWARateMax_vVehSpd/1 -> kph To mps/1, Saturation3/1
  MATLAB Function/1(SWARmax) -> SWARMax_dphiSWARMax/1
  LKA_StrRatio_C/1 -> MATLAB Function/3(i)
  LKA_WhlBaseL_C/1 -> MATLAB Function/4(L)
  kph To mps/1 -> MATLAB Function/1(v)

== system LKAS_AutoSave_DF_20220408_1006_SW62/LKAS/LL/LLOn/LL State Determination (LLStateDet)/LL State Machine Conditions (LLSMCon)/Activation Condition (ActvC) ==
  LKA_Mode : Inport
  bsInInfo : Inport  Port=2
  bsLKAInPInfo : Inport  Port=3
  bsLLClb : Inport  Port=4
  Activation Condition Synthesis (ActvCSyn) : Subsystem  Description=|
      | Block Name: Activation Condition Synthesis
      | Ab.: ActvCSyn
      | No.: 1.1.1.4.4
      | Rev: 0.0.1
      | Update Date: 19-3-26
  Bus Selector : BusSelector  OutputSignals=bsEPSInfo,bsLaneInfo.bsL0Info.L0_Q,bsLaneInfo.bsR0Info.R0_Q
  Bus Selector1 : BusSelector  OutputSignals=LaneWidth,bsDvtInfo.ILftDvt,bsDvtInfo.IRgtDvt
  Deviation Threshold Condition (DvtThresCon) : Subsystem
  EPS Controllability Enable Condition (EPSCtlEC) : Subsystem  Description=|
      | Block Name: EPS Controllability Enable Condition
      | Ab.: EPSCtlEC
      | No.: 1.1.1.4.1
      | Rev: 0.0.1
      | Update Date: 19-3-26
  Lane Quality Enable Condition (LaneQlEC) : Subsystem  Description=|
      | Block Name: Lane Quality Enable Condition
      | Ab.: LaneQlEC
      | No.: 1.1.1.4.3
      | Rev: 0.0.1
      | Update Date: 19-3-26
  stLDWActvCSyn : Outport
  stLKAActvCSyn : Outport  Port=2
  wires:
  [LKA_Mode] -> Activation Condition Synthesis (ActvCSyn)/1(LKA_Mode)
  LKA_Mode/1 -> [LKA_Mode]
  Bus Selector1/1 -> Deviation Threshold Condition (DvtThresCon)/1(DvtThresCon_lLaneWidth)  "<LaneWidth>"
  Bus Selector1/3 -> Deviation Threshold Condition (DvtThresCon)/3(DvtThresCon_IRgtDvt)  "<IRgtDvt>"
  Bus Selector1/2 -> Deviation Threshold Condition (DvtThresCon)/2(DvtThresCon_ILftDvt)  "<ILftDvt>"
  bsLKAInPInfo/1 -> Deviation Threshold Condition (DvtThresCon)/5(DvtThresCon_LKAInfoSyn), Bus Selector1/1
  Deviation Threshold Condition (DvtThresCon)/1(stDvtThresActvFlgLDW) -> Activation Condition Synthesis (ActvCSyn)/3(stDvtThresActvFlgLDW)
  bsLLClb/1 -> Lane Quality Enable Condition (LaneQlEC)/2(LaneQlEC_SingleLane_Disable_Swt), Deviation Threshold Condition (DvtThresCon)/4(DvtThresCon_bsDvtThresClb)
  Activation Condition Synthesis (ActvCSyn)/2(stLKAActvCSyn) -> stLKAActvCSyn/1  "stLKAActvCSyn"
  Lane Quality Enable Condition (LaneQlEC)/1(stLaneQlECFlg) -> Activation Condition Synthesis (ActvCSyn)/5(stLaneQlECFlg)
  EPS Controllability Enable Condition (EPSCtlEC)/1(stEPSCtlEC) -> Activation Condition Synthesis (ActvCSyn)/2(stEPSCtlEC)
  Bus Selector/3 -> Lane Quality Enable Condition (LaneQlEC)/5(LaneQlEC_stFacmR0Ql)  "<R0_Q>"
  Bus Selector/2 -> Lane Quality Enable Condition (LaneQlEC)/4(LaneQlEC_stFacmL0Ql)  "<L0_Q>"
  Bus Selector/1 -> EPS Controllability Enable Condition (EPSCtlEC)/1(EPSCtlEC_bsEPSInfo)  "<bsEPSInfo>"
  Deviation Threshold Condition (DvtThresCon)/2(stDvtThresActvFlgLKA) -> Lane Quality Enable Condition (LaneQlEC)/3(LaneQlEC_stDvtThresActvFlg), Activation Condition Synthesis (ActvCSyn)/4(stDvtThresActvFlgLKA)
  Activation Condition Synthesis (ActvCSyn)/1(stLDWActvCSyn) -> stLDWActvCSyn/1  "stLDWActvCSyn"
  bsInInfo/1 -> Lane Quality Enable Condition (LaneQlEC)/1(LaneQlEC_InInfoSyn), Bus Selector/1

== system LKAS_AutoSave_DF_20220408_1006_SW62/LKAS/LL/LLOn/LL State Determination (LLStateDet)/LL State Machine Conditions (LLSMCon)/Deactivation Condition (DeactvC) ==
  LKA_Mode : Inport
  bsInInfo : Inport  Port=2
  bsLKAInPInfo : Inport  Port=3
  bsLLClb : Inport  Port=4
  LLState : Inport  Port=5
  ExitFlg : Inport  Port=6
  Bus Selector : BusSelector  OutputSignals=bsVehMovInfo.ESC_VehSpd,bsEPSInfo
  Bus Selector1 : BusSelector  OutputSignals=LaneWidth,bsDvtInfo.ILftDvt,bsDvtInfo.IRgtDvt,bsPrCrvtInfo.crPrvwCrvt
  Deactivation Condition Synthesis (DeactvCSyn) : Subsystem  Description=|
      | Block Name: Deactivation Condition Synthesis
      | Ab.: DeactvCSyn
      | No.: 1.1.1.5.3
      | Rev: 0.0.1
      | Update Date: 19-3-26
  Deviation Threshold Condition (DvtThresCon) : Subsystem
  Driver Take Condition (DvrTkCon) : Subsystem  Description=|
      | Block Name: EPS Condition
      | Ab.: EPSC
      | No.: 1.1.1.5.2
      | Rev: 0.0.1
      | Update Date: 19-3-26
  EPS Condition (EPSC) : Subsystem  Description=|
      | Block Name: EPS Condition
      | Ab.: EPSC
      | No.: 1.1.1.5.2
      | Rev: 0.0.1
      | Update Date: 19-3-26
  stLDWDeactvCSyn : Outport
  stLKADeactvCSyn : Outport  Port=2
  wires:
  Deviation Threshold Condition (DvtThresCon)/1(stDvtThresActvFlgLDW) -> Deactivation Condition Synthesis (DeactvCSyn)/2(stDvtThresActvFlgLDW)
  Bus Selector1/1 -> Deviation Threshold Condition (DvtThresCon)/1(LaneWidth)  "<LaneWidth>"
  Bus Selector1/4 -> Driver Take Condition (DvrTkCon)/1(crPrvwCrvt)  "<crPrvwCrvt>"
  Bus Selector1/2 -> Deviation Threshold Condition (DvtThresCon)/2(ILftDvt)  "<ILftDvt>"
  Bus Selector1/3 -> Deviation Threshold Condition (DvtThresCon)/3(IRgtDvt)  "<IRgtDvt>"
  bsLKAInPInfo/1 -> Bus Selector1/1, Deviation Threshold Condition (DvtThresCon)/5(LKAInPInfo)
  Driver Take Condition (DvrTkCon)/1(stDvrTkConFlg) -> Deactivation Condition Synthesis (DeactvCSyn)/4(stDvrTkConFlg)
  Bus Selector/1 -> Driver Take Condition (DvrTkCon)/4(ESC_VehSpd)  "<ESC_VehSpd>"
  Deactivation Condition Synthesis (DeactvCSyn)/2(stLKADeactvCSyn) -> stLKADeactvCSyn/1  "stLKADeactvCSyn"
  LKA_Mode/1 -> Deactivation Condition Synthesis (DeactvCSyn)/1(LKAMode)
  ExitFlg/1 -> Deactivation Condition Synthesis (DeactvCSyn)/6(ExitFlg)
  EPS Condition (EPSC)/1(EPSC_stEPSCFlg) -> Deactivation Condition Synthesis (DeactvCSyn)/5(EPSC_stEPSCFlg)
  Bus Selector/2 -> Driver Take Condition (DvrTkCon)/5(bsEPSInfo), EPS Condition (EPSC)/2(bsEPSInfo)  "<bsEPSInfo>"
  LLState/1 -> EPS Condition (EPSC)/3(LLState)
  Deviation Threshold Condition (DvtThresCon)/2(stDvtThresActvFlgLKA) -> Driver Take Condition (DvrTkCon)/2(DvtThresCon_stDvtThresActvFlgLKA), Deactivation Condition Synthesis (DeactvCSyn)/3(stDvtThresActvFlgLKA)
  bsLLClb/1 -> EPS Condition (EPSC)/1(LLClb), Driver Take Condition (DvrTkCon)/3(LLClb), Deviation Threshold Condition (DvtThresCon)/4(LLClb)
  Deactivation Condition Synthesis (DeactvCSyn)/1(stLDWDeactvCSyn) -> stLDWDeactvCSyn/1
  bsInInfo/1 -> Bus Selector/1

== system LKAS_AutoSave_DF_20220408_1006_SW62/LKAS/LL/LLOn/LL State Determination (LLStateDet)/LL State Machine Conditions (LLSMCon)/Disable Condition (DisblC) ==
  LKA_Mode : Inport
  bsInInfo : Inport  Port=2
  bsLKAInPInfo : Inport  Port=3
  bsLLClb : Inport  Port=4
  LLState : Inport  Port=5
  Disable Condition Synthesis (DisblCSyn) : Subsystem  Description=|
      | Block Name: Disable Condition Synthesis
      | Ab.: DisblCSyn
      | No.: 1.1.1.3.8.0
      | Rev: 0.0.1
      | Update Date: 19-3-26
  Driver Intent Condition (DrvInttC) : Subsystem  Description=|
      | Block Name: Driver Intent Condition
      | Ab.: DrvInttC
      | No.: 1.1.1.3.3.0
      | Rev: 0.0.1
      | Update Date: 19-3-26
  LDW Alarm Timeout (LDWAlrmTOut) : Subsystem  Description=|
      | Block Name: LDW Alarm Timeout
      | Ab.: LDWAlrmTOut
      | No.: 1.1.1.3.6.0
      | Rev: 0.0.1
      | Update Date: 19-3-26
  LDW Own Condition (LDWOwnC) : Subsystem  Description=|
      | Block Name: LDW Own Condition
      | Ab.: LDWOwnC
      | No.: 1.1.1.3.4.0
      | Rev: 0.0.1
      | Update Date: 19-3-26
  LKA Own Condition (LKAOwnC) : Subsystem  Description=|
      | Block Name: LKA Own Condition
      | Ab.: LKAOwnC
      | No.: 1.1.1.3.5.0
      | Rev: 0.0.1
      | Update Date: 19-3-26
  Lane Condition (LaneC) : Subsystem  Description=|
      | Block Name: Lane Condition
      | Ab.: LaneC
      | No.: 1.1.1.3.2.0
      | Rev: 0.0.1
      | Update Date: 19-3-26
  Subsystem : Subsystem  Commented=on
  Subsystem1 : Subsystem
  Vehicle State Condition (VehStateC) : Subsystem  Description=|
      | Block Name: Vehicle State Condition
      | Ab.: VehStateC
      | No.: 1.1.1.3.1.0
      | Rev: 0.0.1
      | Update Date: 19-3-26
  stLDWDisblCSyn : Outport
  stLKADisblCSyn : Outport  Port=2
  Disable_Reason : Outport  Port=3
  wires:
  LDW Own Condition (LDWOwnC)/2(LDWOwnCSyn) -> [LDWOwnCSyn]  "LDWOwnCSyn"
  [LKAInPInfo] -> LKA Own Condition (LKAOwnC)/3(LKAInPInfo)  "LKAInPInfo"
  [LKAInPInfo] -> LDW Own Condition (LDWOwnC)/2(LKAInPInfo)  "LKAInPInfo"
  [LKAInPInfo] -> Driver Intent Condition (DrvInttC)/3(LKAInPInfo)  "LKAInPInfo"
  [LKAInPInfo] -> Lane Condition (LaneC)/2(LKAInPInfo)  "LKAInPInfo"
  bsLKAInPInfo/1 -> [LKAInPInfo]
  [InInfoSyn] -> LKA Own Condition (LKAOwnC)/2(InInfoSyn)  "InInfoSyn"
  [InInfoSyn] -> Driver Intent Condition (DrvInttC)/1(DrvInttC_bsInInfoSyn)  "InInfoSyn"
  [InInfoSyn] -> Lane Condition (LaneC)/1(InInfoSyn)  "InInfoSyn"
  [InInfoSyn] -> Vehicle State Condition (VehStateC)/2(InInfoSyn)  "InInfoSyn"
  bsInInfo/1 -> [InInfoSyn]
  [LLState] -> LDW Alarm Timeout (LDWAlrmTOut)/1(LDWAlrmTOut_bsLLState)
  [LLState] -> LKA Own Condition (LKAOwnC)/4(LLState)  "LLState"
  [LLState] -> Vehicle State Condition (VehStateC)/4(LLState)  "LLState"
  LLState/1 -> [LLState]
  [LLClb] -> LDW Alarm Timeout (LDWAlrmTOut)/2(LDWAlrmTOut_bsLLClb)
  [LLClb] -> LKA Own Condition (LKAOwnC)/5(LLClb)  "LLClb"
  [LLClb] -> LDW Own Condition (LDWOwnC)/3(LLClb)  "LLClb"
  [LLClb] -> Driver Intent Condition (DrvInttC)/2(DrvInttC_bsLLClb)  "LLClb"
  [LLClb] -> Lane Condition (LaneC)/3(LLClb)  "LLClb"
  [LLClb] -> Vehicle State Condition (VehStateC)/3(LLClb)  "LLClb"
  bsLLClb/1 -> [LLClb]
  [VehStateC] -> Subsystem1/1(VehStateC)
  [LaneCSyn] -> Subsystem1/2(LaneCSyn)
  [LKAOwnCSyn] -> Subsystem1/5(LKAOwnCSyn)
  [LDWOwnCSyn] -> Subsystem1/4(LDWOwnCSyn)
  [DrvInttCSyn] -> Subsystem1/3(DrvInttCSyn)
  [LDWAlrmTOutSyn] -> Subsystem1/6(LDWAlrmTOut)
  LDW Alarm Timeout (LDWAlrmTOut)/2(LDWAlrmTOutSyn) -> [LDWAlrmTOutSyn]  "LDWAlrmTOutSyn"
  [stLDWAlrmTOut] -> Disable Condition Synthesis (DisblCSyn)/6(stLDWAlrmTOut)
  [stLDWOwnC] -> Disable Condition Synthesis (DisblCSyn)/5(stLDWOwnC)
  [stLKAOwnC] -> Disable Condition Synthesis (DisblCSyn)/7(stLKAOwnC)
  [stDrvInttC] -> Disable Condition Synthesis (DisblCSyn)/4(stDrvInttC)
  [stLaneC] -> Disable Condition Synthesis (DisblCSyn)/3(stLaneC)
  [stVehStateC] -> Disable Condition Synthesis (DisblCSyn)/2(stVehStateC)
  LKA Own Condition (LKAOwnC)/1(stLKAOwnC) -> [stLKAOwnC]  "stLKAOwnC"
  Driver Intent Condition (DrvInttC)/1(stDrvInttC) -> [stDrvInttC]  "stDrvInttC"
  Lane Condition (LaneC)/1(stLaneC) -> [stLaneC]  "stLaneC"
  [LKA_Mode] -> LKA Own Condition (LKAOwnC)/1(LKA_Mode)  "LKA_Mode"
  [LKA_Mode] -> LDW Own Condition (LDWOwnC)/1(LKA_Mode)  "LKA_Mode"
  [LKA_Mode] -> Vehicle State Condition (VehStateC)/1(LKA_Mode)  "LKA_Mode"
  [LKA_Mode] -> Disable Condition Synthesis (DisblCSyn)/1(LKA_Mode)  "LKA_Mode"
  LKA_Mode/1 -> [LKA_Mode]
  Subsystem1/1(DisableReason) -> Disable_Reason/1  "Disable_Reason"
  Vehicle State Condition (VehStateC)/2(VehStateC) -> [VehStateC]  "VehStateC"
  Lane Condition (LaneC)/2(LaneCSyn) -> [LaneCSyn]  "LaneCSyn"
  Driver Intent Condition (DrvInttC)/2(DrvInttCSyn) -> [DrvInttCSyn]  "DrvInttCSyn"
  LKA Own Condition (LKAOwnC)/2(LKAOwnCSyn) -> [LKAOwnCSyn]  "LKAOwnCSyn"
  Disable Condition Synthesis (DisblCSyn)/2(stLKADisblCSyn) -> stLKADisblCSyn/1  "stLKADisblCSyn"
  LDW Alarm Timeout (LDWAlrmTOut)/1(stLDWAlrmTOut) -> [stLDWAlrmTOut]  "stLDWAlrmTOut"
  Disable Condition Synthesis (DisblCSyn)/1(stLDWDisblCSyn) -> stLDWDisblCSyn/1  "stLDWDisblCSyn"
  LDW Own Condition (LDWOwnC)/1(stLDWOwnC) -> [stLDWOwnC]  "stLDWOwnC"
  Vehicle State Condition (VehStateC)/1(stVehStateC) -> [stVehStateC]  "stVehStateC"

== system LKAS_AutoSave_DF_20220408_1006_SW62/LKAS/LL/LLOn/LL State Determination (LLStateDet)/LL State Machine Conditions (LLSMCon)/Enable Condition (EnaC) ==
  LKA_Mode : Inport
  bsInInfo : Inport  Port=2
  bsLKAInPInfo : Inport  Port=3
  bsLLClb : Inport  Port=4
  Driver Intent Condition (DrvInttC) : Subsystem  Description=|
      | Block Name: Driver Intent Condition
      | Ab.: DrvInttC
      | No.: 1.1.1.2.3.0
      | Rev: 0.0.1
      | Update Date: 19-3-26
  Enable Condition Synthesis (EnaCSyn) : Subsystem  Description=|
      | Block Name: Enable Condition Synthesis
      | Ab.: EnaCSyn
      | No.: 1.1.1.2.7.0
      | Rev: 0.0.1
      | Update Date: 19-3-26
  LDW Own Condition (LDWOwnC) : Subsystem  Description=|
      | Block Name: LDW Own Condition
      | Ab.: LDWOwnC
      | No.: 1.1.1.2.4.0
      | Rev: 0.0.1
      | Update Date: 19-3-26
  LKA Own Condition (LKAOwnC) : Subsystem  Description=|
      | Block Name: LKA Own Condition
      | Ab.: LKAOwnC
      | No.: 1.1.1.2.5.0
      | Rev: 0.0.1
      | Update Date: 19-3-26
  Lane Condition (LaneC) : Subsystem  Description=|
      | Block Name: Lane Condition
      | Ab.: LaneC
      | No.: 1.1.1.2.2.0
      | Rev: 0.0.1
      | Update Date: 19-3-26
  Vehicle State Condition (VehStateC) : Subsystem  Description=|
      | Block Name: Vehicle State Condition
      | Ab.: VehStateC
      | No.: 1.1.1.2.1.0
      | Rev: 0.0.1
      | Update Date: 19-3-26
  stLDWEnaCSyn : Outport
  stLKAEnaCSyn : Outport  Port=2
  wires:
  [LKA_Mode] -> LKA Own Condition (LKAOwnC)/1(LKA_Mode)
  [LKAInPInfo] -> LKA Own Condition (LKAOwnC)/3(LKAInPInfo)
  [LKAInPInfo] -> LDW Own Condition (LDWOwnC)/2(LKAInPInfo)
  [LKA_Mode] -> LDW Own Condition (LDWOwnC)/1(LKA_Mode)
  [LKAInPInfo] -> Lane Condition (LaneC)/2(LKAInPInfo)
  [LLClb] -> LKA Own Condition (LKAOwnC)/4(LLClb)
  [LLClb] -> LDW Own Condition (LDWOwnC)/3(LLClb)
  [LLClb] -> Driver Intent Condition (DrvInttC)/2(LLClb)
  [LLClb] -> Lane Condition (LaneC)/3(LLClb)
  [LLClb] -> Vehicle State Condition (VehStateC)/3(LLClb)
  [InInfoSyn] -> LKA Own Condition (LKAOwnC)/2(InInfoSyn)
  [InInfoSyn] -> Driver Intent Condition (DrvInttC)/1(InInfoSyn)
  [InInfoSyn] -> Lane Condition (LaneC)/1(InInfoSyn)
  [InInfoSyn] -> Vehicle State Condition (VehStateC)/2(InInfoSyn)
  bsLLClb/1 -> [LLClb]  "LLClb"
  bsLKAInPInfo/1 -> [LKAInPInfo]  "LKAInPInfo"
  bsInInfo/1 -> [InInfoSyn]  "InInfoSyn"
  LKA Own Condition (LKAOwnC)/1(stLKAOwnC) -> [stLKAOwnC]  "stLKAOwnC"
  LDW Own Condition (LDWOwnC)/1(stLDWOwnC) -> [stLDWOwnC]  "stLDWOwnC"
  Driver Intent Condition (DrvInttC)/1(stDrvInttC) -> [stDrvInttC]  "stDrvInttC"
  Lane Condition (LaneC)/1(stLaneC) -> [stLaneC]  "stLaneC"
  Vehicle State Condition (VehStateC)/1(stVehStateC) -> [stVehStateC]
  [stLDWOwnC] -> Enable Condition Synthesis (EnaCSyn)/5(stLDWOwnC)
  [stLKAOwnC] -> Enable Condition Synthesis (EnaCSyn)/6(stLKAOwnC)
  [stDrvInttC] -> Enable Condition Synthesis (EnaCSyn)/4(stDrvInttC)
  [stLaneC] -> Enable Condition Synthesis (EnaCSyn)/3(stLaneC)
  [stVehStateC] -> Enable Condition Synthesis (EnaCSyn)/2(stVehStateC)
  [LKA_Mode] -> Vehicle State Condition (VehStateC)/1(LKA_Mode)
  [LKA_Mode] -> Enable Condition Synthesis (EnaCSyn)/1(LKA_Mode)  "LKA_Mode"
  Enable Condition Synthesis (EnaCSyn)/2(stLKAEnaCSyn) -> stLKAEnaCSyn/1  "stLKAEnaCSyn"
  LKA_Mode/1 -> [LKA_Mode]
  Enable Condition Synthesis (EnaCSyn)/1(stLDWEnaCSyn) -> stLDWEnaCSyn/1  "stLDWEnaCSyn"
